simulink library "sm_ratchet_pawl_lib"  (R2025a)
settings: Solver=VariableStepAuto  StartTime=0.0  StopTime=10.0  RelTol=1e-3
undefined symbols (not defined in the file): contact_WR, G1a, G1b, G2a, G2b, G3a, G3b, G4a, G4b, G5a, G5b, line, X, Y, Z
libraries: sm_lib x12, $bdroot x10
Description:
  | Copyright 2024-2026 The MathWorks, Inc.
settings Model: Creator=smiller  LastModifiedBy=smiller
settings RTWCC: GPUComputeCapability=3.5

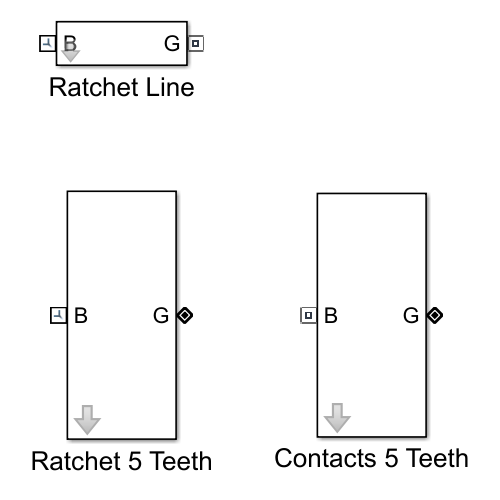
[thumbnail: Simulink's stored preview of the top-level diagram]
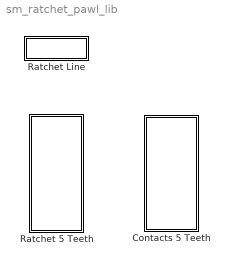
== system sm_ratchet_pawl_lib ==
  Contacts 5 Teeth : Subsystem  mask{k_whl=contact_WR.k, b_whl=contact_WR.b, x_whl=contact_WR.x, s_whl=contact_WR.s, d_whl=contact_WR.d, v_whl=contact_WR.v}
      mask prompts: k_whl "Stiffness"; b_whl "Damping"; x_whl "Transition Width"; s_whl "Friction Static"; d_whl "Friction Dynamic"; v_whl "Velocity Threshold"
  Ratchet 5 Teeth : Subsystem  mask{ind_set=0}
      mask prompts: ind_set "Line Index (2 per tooth)"
  Ratchet Line : Subsystem  mask{ind=1}
      mask prompts: ind "Line Index"

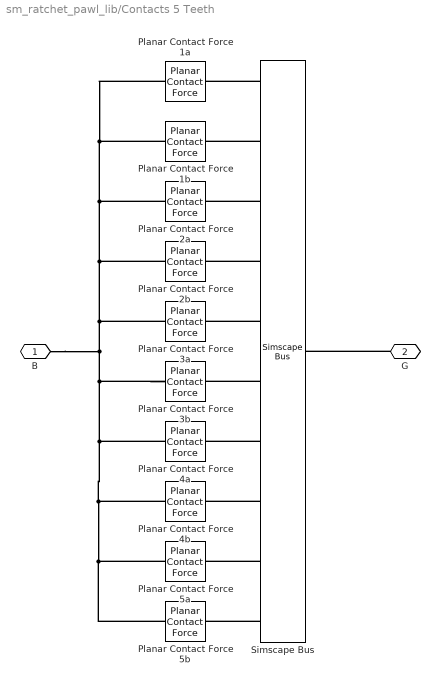
== system sm_ratchet_pawl_lib/Contacts 5 Teeth ==
  Planar Contact Force 1a : sm_lib/Forces and Torques/Planar Contact Force  NormalForceType=SmoothSpringDamper  NormalStiffness=k_whl  NormalStiffnessUnits=N/m  NormalDamping=b_whl  NormalDampingUnits=N/(m/s)  NormalTransitionRegionWidth=x_whl  NormalTransitionRegionWidthUnits=m  FrictionType=SmoothStickSlip  CoefficientOfStaticFriction=x_whl  CoefficientOfDynamicFriction=d_whl  FrictionalCriticalVelocity=v_whl  FrictionalCriticalVelocityUnits=m/s  SenseContactSignal=off  SensePenetrationDepth=off  SenseNormalVelocity=off  SenseTangentialVelocity=off  SensingForceTorqueDirection=BaseOnFollower  SensingForceTorqueResolutionFrame=ContactFrame  SenseNormalForce=off  SenseNormalForceMagnitude=off  SenseNormalTorque=off  SenseFrictionalForce=off  SenseFrictionalForceMagnitude=off  SenseFrictionalTorque=off  SenseTotalForce=off  SenseTotalTorque=off  SenseContactBaseRotation=off  SenseContactBaseTranslation=off  SenseContactFollowerRotation=off  SenseContactFollowerTranslation=off  ZeroCrossDetectContactStartAndEnd=on
  Planar Contact Force 1b : sm_lib/Forces and Torques/Planar Contact Force  NormalForceType=SmoothSpringDamper  NormalStiffness=k_whl  NormalStiffnessUnits=N/m  NormalDamping=b_whl  NormalDampingUnits=N/(m/s)  NormalTransitionRegionWidth=x_whl  NormalTransitionRegionWidthUnits=m  FrictionType=SmoothStickSlip  CoefficientOfStaticFriction=x_whl  CoefficientOfDynamicFriction=d_whl  FrictionalCriticalVelocity=v_whl  FrictionalCriticalVelocityUnits=m/s  SenseContactSignal=off  SensePenetrationDepth=off  SenseNormalVelocity=off  SenseTangentialVelocity=off  SensingForceTorqueDirection=BaseOnFollower  SensingForceTorqueResolutionFrame=ContactFrame  SenseNormalForce=off  SenseNormalForceMagnitude=off  SenseNormalTorque=off  SenseFrictionalForce=off  SenseFrictionalForceMagnitude=off  SenseFrictionalTorque=off  SenseTotalForce=off  SenseTotalTorque=off  SenseContactBaseRotation=off  SenseContactBaseTranslation=off  SenseContactFollowerRotation=off  SenseContactFollowerTranslation=off  ZeroCrossDetectContactStartAndEnd=on
  Planar Contact Force 2a : sm_lib/Forces and Torques/Planar Contact Force  NormalForceType=SmoothSpringDamper  NormalStiffness=k_whl  NormalStiffnessUnits=N/m  NormalDamping=b_whl  NormalDampingUnits=N/(m/s)  NormalTransitionRegionWidth=x_whl  NormalTransitionRegionWidthUnits=m  FrictionType=SmoothStickSlip  CoefficientOfStaticFriction=x_whl  CoefficientOfDynamicFriction=d_whl  FrictionalCriticalVelocity=v_whl  FrictionalCriticalVelocityUnits=m/s  SenseContactSignal=off  SensePenetrationDepth=off  SenseNormalVelocity=off  SenseTangentialVelocity=off  SensingForceTorqueDirection=BaseOnFollower  SensingForceTorqueResolutionFrame=ContactFrame  SenseNormalForce=off  SenseNormalForceMagnitude=off  SenseNormalTorque=off  SenseFrictionalForce=off  SenseFrictionalForceMagnitude=off  SenseFrictionalTorque=off  SenseTotalForce=off  SenseTotalTorque=off  SenseContactBaseRotation=off  SenseContactBaseTranslation=off  SenseContactFollowerRotation=off  SenseContactFollowerTranslation=off  ZeroCrossDetectContactStartAndEnd=on
  Planar Contact Force 2b : sm_lib/Forces and Torques/Planar Contact Force  NormalForceType=SmoothSpringDamper  NormalStiffness=k_whl  NormalStiffnessUnits=N/m  NormalDamping=b_whl  NormalDampingUnits=N/(m/s)  NormalTransitionRegionWidth=x_whl  NormalTransitionRegionWidthUnits=m  FrictionType=SmoothStickSlip  CoefficientOfStaticFriction=x_whl  CoefficientOfDynamicFriction=d_whl  FrictionalCriticalVelocity=v_whl  FrictionalCriticalVelocityUnits=m/s  SenseContactSignal=off  SensePenetrationDepth=off  SenseNormalVelocity=off  SenseTangentialVelocity=off  SensingForceTorqueDirection=BaseOnFollower  SensingForceTorqueResolutionFrame=ContactFrame  SenseNormalForce=off  SenseNormalForceMagnitude=off  SenseNormalTorque=off  SenseFrictionalForce=off  SenseFrictionalForceMagnitude=off  SenseFrictionalTorque=off  SenseTotalForce=off  SenseTotalTorque=off  SenseContactBaseRotation=off  SenseContactBaseTranslation=off  SenseContactFollowerRotation=off  SenseContactFollowerTranslation=off  ZeroCrossDetectContactStartAndEnd=on
  Planar Contact Force 3a : sm_lib/Forces and Torques/Planar Contact Force  NormalForceType=SmoothSpringDamper  NormalStiffness=k_whl  NormalStiffnessUnits=N/m  NormalDamping=b_whl  NormalDampingUnits=N/(m/s)  NormalTransitionRegionWidth=x_whl  NormalTransitionRegionWidthUnits=m  FrictionType=SmoothStickSlip  CoefficientOfStaticFriction=x_whl  CoefficientOfDynamicFriction=d_whl  FrictionalCriticalVelocity=v_whl  FrictionalCriticalVelocityUnits=m/s  SenseContactSignal=off  SensePenetrationDepth=off  SenseNormalVelocity=off  SenseTangentialVelocity=off  SensingForceTorqueDirection=BaseOnFollower  SensingForceTorqueResolutionFrame=ContactFrame  SenseNormalForce=off  SenseNormalForceMagnitude=off  SenseNormalTorque=off  SenseFrictionalForce=off  SenseFrictionalForceMagnitude=off  SenseFrictionalTorque=off  SenseTotalForce=off  SenseTotalTorque=off  SenseContactBaseRotation=off  SenseContactBaseTranslation=off  SenseContactFollowerRotation=off  SenseContactFollowerTranslation=off  ZeroCrossDetectContactStartAndEnd=on
  Planar Contact Force 3b : sm_lib/Forces and Torques/Planar Contact Force  NormalForceType=SmoothSpringDamper  NormalStiffness=k_whl  NormalStiffnessUnits=N/m  NormalDamping=b_whl  NormalDampingUnits=N/(m/s)  NormalTransitionRegionWidth=x_whl  NormalTransitionRegionWidthUnits=m  FrictionType=SmoothStickSlip  CoefficientOfStaticFriction=x_whl  CoefficientOfDynamicFriction=d_whl  FrictionalCriticalVelocity=v_whl  FrictionalCriticalVelocityUnits=m/s  SenseContactSignal=off  SensePenetrationDepth=off  SenseNormalVelocity=off  SenseTangentialVelocity=off  SensingForceTorqueDirection=BaseOnFollower  SensingForceTorqueResolutionFrame=ContactFrame  SenseNormalForce=off  SenseNormalForceMagnitude=off  SenseNormalTorque=off  SenseFrictionalForce=off  SenseFrictionalForceMagnitude=off  SenseFrictionalTorque=off  SenseTotalForce=off  SenseTotalTorque=off  SenseContactBaseRotation=off  SenseContactBaseTranslation=off  SenseContactFollowerRotation=off  SenseContactFollowerTranslation=off  ZeroCrossDetectContactStartAndEnd=on
  Planar Contact Force 4a : sm_lib/Forces and Torques/Planar Contact Force  NormalForceType=SmoothSpringDamper  NormalStiffness=k_whl  NormalStiffnessUnits=N/m  NormalDamping=b_whl  NormalDampingUnits=N/(m/s)  NormalTransitionRegionWidth=x_whl  NormalTransitionRegionWidthUnits=m  FrictionType=SmoothStickSlip  CoefficientOfStaticFriction=x_whl  CoefficientOfDynamicFriction=d_whl  FrictionalCriticalVelocity=v_whl  FrictionalCriticalVelocityUnits=m/s  SenseContactSignal=off  SensePenetrationDepth=off  SenseNormalVelocity=off  SenseTangentialVelocity=off  SensingForceTorqueDirection=BaseOnFollower  SensingForceTorqueResolutionFrame=ContactFrame  SenseNormalForce=off  SenseNormalForceMagnitude=off  SenseNormalTorque=off  SenseFrictionalForce=off  SenseFrictionalForceMagnitude=off  SenseFrictionalTorque=off  SenseTotalForce=off  SenseTotalTorque=off  SenseContactBaseRotation=off  SenseContactBaseTranslation=off  SenseContactFollowerRotation=off  SenseContactFollowerTranslation=off  ZeroCrossDetectContactStartAndEnd=on
  Planar Contact Force 4b : sm_lib/Forces and Torques/Planar Contact Force  NormalForceType=SmoothSpringDamper  NormalStiffness=k_whl  NormalStiffnessUnits=N/m  NormalDamping=b_whl  NormalDampingUnits=N/(m/s)  NormalTransitionRegionWidth=x_whl  NormalTransitionRegionWidthUnits=m  FrictionType=SmoothStickSlip  CoefficientOfStaticFriction=x_whl  CoefficientOfDynamicFriction=d_whl  FrictionalCriticalVelocity=v_whl  FrictionalCriticalVelocityUnits=m/s  SenseContactSignal=off  SensePenetrationDepth=off  SenseNormalVelocity=off  SenseTangentialVelocity=off  SensingForceTorqueDirection=BaseOnFollower  SensingForceTorqueResolutionFrame=ContactFrame  SenseNormalForce=off  SenseNormalForceMagnitude=off  SenseNormalTorque=off  SenseFrictionalForce=off  SenseFrictionalForceMagnitude=off  SenseFrictionalTorque=off  SenseTotalForce=off  SenseTotalTorque=off  SenseContactBaseRotation=off  SenseContactBaseTranslation=off  SenseContactFollowerRotation=off  SenseContactFollowerTranslation=off  ZeroCrossDetectContactStartAndEnd=on
  Planar Contact Force 5a : sm_lib/Forces and Torques/Planar Contact Force  NormalForceType=SmoothSpringDamper  NormalStiffness=k_whl  NormalStiffnessUnits=N/m  NormalDamping=b_whl  NormalDampingUnits=N/(m/s)  NormalTransitionRegionWidth=x_whl  NormalTransitionRegionWidthUnits=m  FrictionType=SmoothStickSlip  CoefficientOfStaticFriction=x_whl  CoefficientOfDynamicFriction=d_whl  FrictionalCriticalVelocity=v_whl  FrictionalCriticalVelocityUnits=m/s  SenseContactSignal=off  SensePenetrationDepth=off  SenseNormalVelocity=off  SenseTangentialVelocity=off  SensingForceTorqueDirection=BaseOnFollower  SensingForceTorqueResolutionFrame=ContactFrame  SenseNormalForce=off  SenseNormalForceMagnitude=off  SenseNormalTorque=off  SenseFrictionalForce=off  SenseFrictionalForceMagnitude=off  SenseFrictionalTorque=off  SenseTotalForce=off  SenseTotalTorque=off  SenseContactBaseRotation=off  SenseContactBaseTranslation=off  SenseContactFollowerRotation=off  SenseContactFollowerTranslation=off  ZeroCrossDetectContactStartAndEnd=on
  Planar Contact Force 5b : sm_lib/Forces and Torques/Planar Contact Force  NormalForceType=SmoothSpringDamper  NormalStiffness=k_whl  NormalStiffnessUnits=N/m  NormalDamping=b_whl  NormalDampingUnits=N/(m/s)  NormalTransitionRegionWidth=x_whl  NormalTransitionRegionWidthUnits=m  FrictionType=SmoothStickSlip  CoefficientOfStaticFriction=x_whl  CoefficientOfDynamicFriction=d_whl  FrictionalCriticalVelocity=v_whl  FrictionalCriticalVelocityUnits=m/s  SenseContactSignal=off  SensePenetrationDepth=off  SenseNormalVelocity=off  SenseTangentialVelocity=off  SensingForceTorqueDirection=BaseOnFollower  SensingForceTorqueResolutionFrame=ContactFrame  SenseNormalForce=off  SenseNormalForceMagnitude=off  SenseNormalTorque=off  SenseFrictionalForce=off  SenseFrictionalForceMagnitude=off  SenseFrictionalTorque=off  SenseTotalForce=off  SenseTotalTorque=off  SenseContactBaseRotation=off  SenseContactBaseTranslation=off  SenseContactFollowerRotation=off  SenseContactFollowerTranslation=off  ZeroCrossDetectContactStartAndEnd=on
  Simscape Bus : SimscapeBus  HierarchyStrings=G1a;G1b;G2a;G2b;G3a;G3b;G4a;G4b;G5a;G5b
  B : PMIOPort  Side=Left
  G : PMIOPort  Port=2  Side=Right
  connections:
  Planar Contact Force 5b/LConn1 -- Planar Contact Force 4b/LConn1 -- Planar Contact Force 4a/LConn1 -- Planar Contact Force 3b/LConn1 -- Planar Contact Force 2a/LConn1 -- Planar Contact Force 1a/LConn1 -- Planar Contact Force 1b/LConn1 -- Planar Contact Force 2b/LConn1 -- Planar Contact Force 3a/LConn1 -- B/RConn1 -- Planar Contact Force 5a/LConn1
  Simscape Bus/LConn1 -- Planar Contact Force 1a/RConn1
  Simscape Bus/LConn2 -- Planar Contact Force 1b/RConn1
  Simscape Bus/LConn3 -- Planar Contact Force 2a/RConn1
  Simscape Bus/LConn4 -- Planar Contact Force 2b/RConn1
  Simscape Bus/LConn5 -- Planar Contact Force 3a/RConn1
  Simscape Bus/LConn10 -- Planar Contact Force 5b/RConn1
  Simscape Bus/LConn9 -- Planar Contact Force 5a/RConn1
  Simscape Bus/LConn8 -- Planar Contact Force 4b/RConn1
  Simscape Bus/LConn6 -- Planar Contact Force 3b/RConn1
  Simscape Bus/LConn7 -- Planar Contact Force 4a/RConn1
  G/RConn1 -- Simscape Bus/RConn1

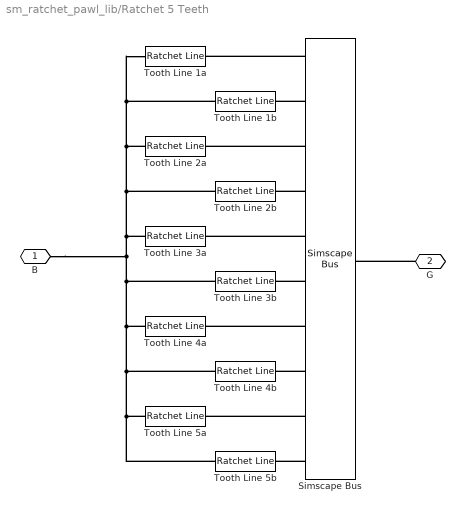
== system sm_ratchet_pawl_lib/Ratchet 5 Teeth ==
  Simscape Bus : SimscapeBus  HierarchyStrings=G1a;G1b;G2a;G2b;G3a;G3b;G4a;G4b;G5a;G5b
  Tooth Line 1a : $bdroot/Ratchet Line  ind=ind_set+1
  Tooth Line 1b : $bdroot/Ratchet Line  ind=ind_set+2
  Tooth Line 2a : $bdroot/Ratchet Line  ind=ind_set+3
  Tooth Line 2b : $bdroot/Ratchet Line  ind=ind_set+4
  Tooth Line 3a : $bdroot/Ratchet Line  ind=ind_set+5
  Tooth Line 3b : $bdroot/Ratchet Line  ind=ind_set+6
  Tooth Line 4a : $bdroot/Ratchet Line  ind=ind_set+7
  Tooth Line 4b : $bdroot/Ratchet Line  ind=ind_set+8
  Tooth Line 5a : $bdroot/Ratchet Line  ind=ind_set+9
  Tooth Line 5b : $bdroot/Ratchet Line  ind=ind_set+10
  B : PMIOPort  Side=Left
  G : PMIOPort  Port=2  Side=Right
  connections:
  Tooth Line 3a/LConn1 -- B/RConn1 -- Tooth Line 5b/LConn1 -- Tooth Line 5a/LConn1 -- Tooth Line 4b/LConn1 -- Tooth Line 4a/LConn1 -- Tooth Line 3b/LConn1 -- Tooth Line 1a/LConn1 -- Tooth Line 1b/LConn1 -- Tooth Line 2a/LConn1 -- Tooth Line 2b/LConn1
  Simscape Bus/LConn1 -- Tooth Line 1a/RConn1
  Simscape Bus/LConn2 -- Tooth Line 1b/RConn1
  Simscape Bus/LConn3 -- Tooth Line 2a/RConn1
  Simscape Bus/LConn4 -- Tooth Line 2b/RConn1
  Simscape Bus/LConn5 -- Tooth Line 3a/RConn1
  Simscape Bus/LConn10 -- Tooth Line 5b/RConn1
  Simscape Bus/LConn9 -- Tooth Line 5a/RConn1
  Simscape Bus/LConn8 -- Tooth Line 4b/RConn1
  Simscape Bus/LConn6 -- Tooth Line 3b/RConn1
  Simscape Bus/LConn7 -- Tooth Line 4a/RConn1
  G/RConn1 -- Simscape Bus/RConn1

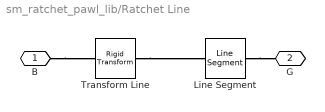
== system sm_ratchet_pawl_lib/Ratchet Line ==
  Line Segment : sm_lib/Curves and Surfaces/Line Segment  Length=line.l(ind)  LengthUnits=m  GraphicType=FromGeometry  GraphicVisPropType=SimpleVisualProperties  GraphicDiffuseColor=[0 0 1]  GraphicOpacity=1.0  GraphicSpecularColor=[0.5 0.5 0.5 1.0]  GraphicAmbientColor=[0.15 0.15 0.15 1.0]  GraphicEmissiveColor=[0.0 0.0 0.0 1.0]  GraphicShininess=75
  Transform Line : sm_lib/Frames and Transforms/Rigid Transform  RotationMethod=RotationSequence  FollAlignAxisA=+X  BaseAlignAxisA=+Y  FollAlignAxisB=+Y  BaseAlignAxisB=+Z  RotationStandardAxis=+Z  RotationAngle=0.0  RotationAngleUnits=deg  RotationArbitraryAxis=[0 0 1]  RotationSequenceAxes=FollowerAxes  RotationSequence=ZXY  RotationSequenceAngles=[line.q(ind) 0 0]  RotationSequenceAnglesUnits=deg  RotationMatrix=[1 0 0; 0 1 0; 0 0 1]  Quaternion=[1 0 0 0]  TranslationMethod=Cartesian  TranslationCartesianOffset=[line.o(ind,:) 0]  TranslationCartesianOffsetUnits=m  TranslationStandardAxis=+Z  TranslationStandardOffset=0  TranslationStandardOffsetUnits=m  TranslationROffset=0  TranslationROffsetUnits=m  TranslationThetaOffset=0  TranslationThetaOffsetUnits=deg  TranslationZOffset=0  TranslationZOffsetUnits=m
  B : PMIOPort  Side=Left
  G : PMIOPort  Port=2  Side=Right
  connections:
  B/RConn1 -- Transform Line/LConn1
  Line Segment/RConn1 -- G/RConn1
  Transform Line/RConn1 -- Line Segment/LConn1
